simulink model "uniciclo_FL_old"  (R2020a)
settings: Solver=VariableStepAuto  StartTime=0.0  StopTime=10.0  RelTol=1e-3
settings Model: Creator=Andrea_Ferroni  LastModifiedBy=Andrea_Ferroni

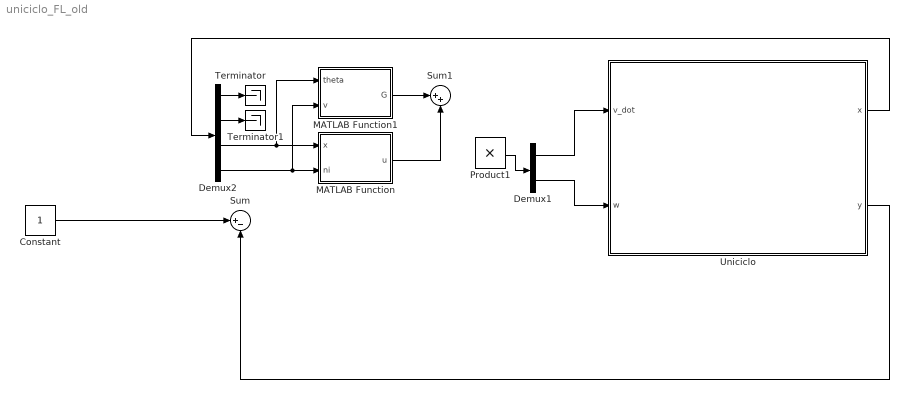
== system uniciclo_FL_old ==
  Constant : Constant
  Demux1 : Demux  Outputs=2
  Demux2 : Demux
  MATLAB Function : MATLAB Function  TreatAsAtomicUnit=on
  MATLAB Function1 : MATLAB Function  TreatAsAtomicUnit=on
  Product1 : Product
  Sum : Sum  Inputs=|+-
  Sum1 : Sum  Inputs=|++
  Terminator : Terminator
  Terminator1 : Terminator
  Uniciclo : Subsystem
  wires:
  Product1/1 -> Demux1/1
  Demux1/1 -> Uniciclo/1(v_dot)
  Demux1/2 -> Uniciclo/2(w)
  Uniciclo/1(x) -> Demux2/1
  Constant/1 -> Sum/1
  Uniciclo/2(y) -> Sum/2
  Demux2/1 -> Terminator/1
  Demux2/2 -> Terminator1/1
  Demux2/3 -> MATLAB Function1/1(theta), MATLAB Function/1(x)
  Demux2/4 -> MATLAB Function1/2(v), MATLAB Function/2(ni)
  MATLAB Function1/1(G) -> Sum1/1
  MATLAB Function/1(u) -> Sum1/2

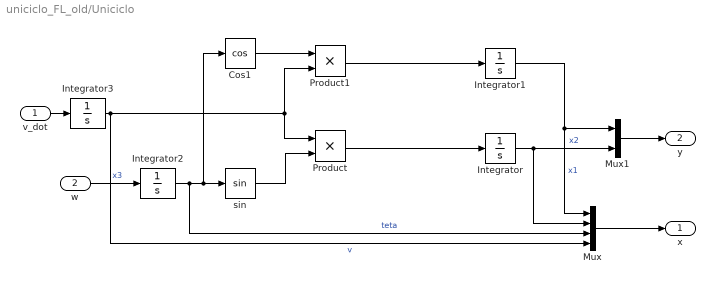
== system uniciclo_FL_old/Uniciclo ==
  v_dot : Inport
  w : Inport  Port=2
  Cos1 : Trigonometry  Operator=cos
  Integrator : Integrator
  Integrator1 : Integrator
  Integrator2 : Integrator  InitialCondition=pi/2
  Integrator3 : Integrator  InitialCondition=pi/2
  Mux : Mux
  Mux1 : Mux  Inputs=2
  Product : Product
  Product1 : Product
  sin : Trigonometry
  x : Outport
  y : Outport  Port=2
  wires:
  v_dot/1 -> Integrator3/1
  Cos1/1 -> Product1/1
  Product1/1 -> Integrator1/1
  Product/1 -> Integrator/1
  w/1 -> Integrator2/1  "x3"
  Integrator2/1 -> Mux/3, Cos1/1, sin/1  "teta"
  sin/1 -> Product/2
  Mux/1 -> x/1
  Integrator1/1 -> Mux/1, Mux1/1  "x1"
  Integrator/1 -> Mux/2, Mux1/2  "x2"
  Mux1/1 -> y/1
  Integrator3/1 -> Mux/4, Product1/2, Product/1  "v"

== matlab function uniciclo_FL_old/MATLAB Function ==
  data: x input; ni input; u output
function u = Linearized(x,ni)
theta = x(3);
v = x(4);
E_inv = inv_E(theta, v);
G = Gamma(theta, v);
u =  -E_inv*G + E_inv*ni;
end

% gamma
function G = Gamma(theta, v)
G = [0;0];
end
% 
function E_inv = inv_E(theta, v)
E = [cos(theta) -v*sin(theta);
	 sin(theta)  v*cos(theta)];
E_inv = inv(E);
end

== matlab function uniciclo_FL_old/MATLAB Function1 ==
  data: theta input; G output; v input
function G = Gamma(theta, v)
G = [0;0];
end
